simulink model "Integrated_Model"  (R2023b)
settings: Solver=ode23s  StartTime=0.0  StopTime=120  FixedStep=0.01  RelTol=1e-3
undefined symbols (not defined in the file): A_sm, A_stack, A_VGS_center, cmp, cp_coolant, ctrl, estNcr, eta_hex, eta_M, J_rotor, k_e_M, k_t_M, lambda, M_H2O, M_Nmix, M_O2, m_st_Nmix_init, m_st_O2_init, m_st_vp_init, p_amb, p_init, R_init, R_M, R_Nmix, R_O2, R_vp, RH_amb, T_amb, T_coolant, T_init, tbn, V_sm, V_stack, V_tbn_m, yO2_amb
libraries: slpidlib x5
(part 2 of 3)

== system Integrated_Model/SimpleFCstack/Calc_outlet_humidity ==
  note: ※凝縮が生じない場合の分圧比はモル分率に等しい
  RHin [-] : Inport
  Tin [K] : Inport  Port=2
  Tout [K] : Inport  Port=3
  pin [Pa] : Inport  Port=4
  pout [Pa] : Inport  Port=5
  Divide : Product  Inputs=*/
  Divide1 : Product  Inputs=*/
  MATLAB Function : MATLAB Function  TreatAsAtomicUnit=on
  MATLAB Function1 : MATLAB Function  TreatAsAtomicUnit=on
  Product : Product
  Product1 : Product
  Terminator : Terminator
  RHout [-] : Outport
  wires:
  MATLAB Function/1(psat) -> Product/2
  Tin [K]/1 -> MATLAB Function/1(Ts)
  Tout [K]/1 -> MATLAB Function1/1(Ts)
  RHin [-]/1 -> Product/1
  Product/1 -> Terminator/1, Divide/1  "pin,vp"
  pin [Pa]/1 -> Divide/2
  Divide/1 -> Product1/1  "pin,vp/pin"
  pout [Pa]/1 -> Product1/2
  Product1/1 -> Divide1/1  "pout,vp"
  MATLAB Function1/1(psat) -> Divide1/2
  Divide1/1 -> RHout [-]/1

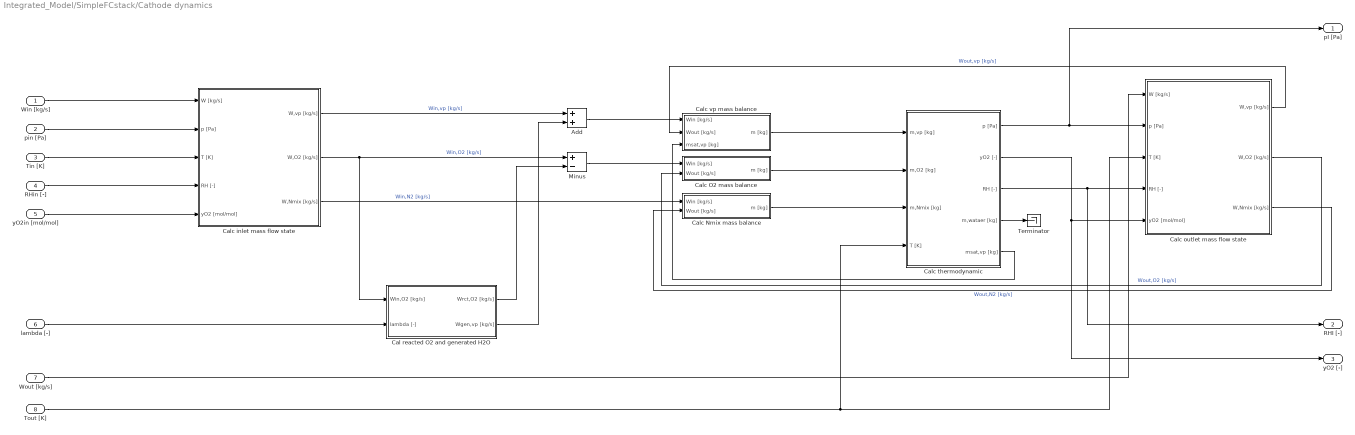
== system Integrated_Model/SimpleFCstack/Cathode dynamics ==
  Win [kg/s] : Inport
  pin [Pa] : Inport  Port=2
  Tin [K] : Inport  Port=3
  RHin [-] : Inport  Port=4
  yO2in [mol/mol] : Inport  Port=5
  lambda [-] : Inport  Port=6
  Wout [kg/s] : Inport  Port=7
  Tout [K] : Inport  Port=8
  Add : Sum
  Cal reacted O2 and generated H2O : Subsystem
  Calc Nmix mass balance : Subsystem
  Calc O2 mass balance : Subsystem
  Calc inlet mass flow state : Subsystem
  Calc outlet mass flow state : Subsystem
  Calc thermodynamic : Subsystem
  Calc vp mass balance : Subsystem
  Minus : Sum  Inputs=+-
  Terminator : Terminator
  pI [Pa] : Outport
  RHI [-] : Outport  Port=2
  yO2 [-] : Outport  Port=3
  wires:
  Calc outlet mass flow state/3(W,Nmix [kg/s]) -> Calc Nmix mass balance/2(Wout [kg/s])  "Wout,N2 [kg/s]"
  Calc vp mass balance/1(m [kg]) -> Calc thermodynamic/1(m,vp [kg])
  RHin [-]/1 -> Calc inlet mass flow state/4(RH [-])
  Calc outlet mass flow state/1(W,vp [kg/s]) -> Calc vp mass balance/2(Wout [kg/s])  "Wout,vp [kg/s]"
  Calc inlet mass flow state/2(W,O2 [kg/s]) -> Minus/1, Cal reacted O2 and generated H2O/1(Win,O2 [kg/s])  "Win,O2 [kg/s]"
  Win [kg/s]/1 -> Calc inlet mass flow state/1(W [kg/s])
  Calc O2 mass balance/1(m [kg]) -> Calc thermodynamic/2(m,O2 [kg])
  lambda [-]/1 -> Cal reacted O2 and generated H2O/2(lambda [-])
  Minus/1 -> Calc O2 mass balance/1(Win [kg/s])
  Calc thermodynamic/2(yO2 [-]) -> yO2 [-]/1, Calc outlet mass flow state/5(yO2 [mol/mol])
  Tout [K]/1 -> Calc outlet mass flow state/3(T [K]), Calc thermodynamic/4(T [K])
  Calc outlet mass flow state/2(W,O2 [kg/s]) -> Calc O2 mass balance/2(Wout [kg/s])  "Wout,O2 [kg/s]"
  Calc inlet mass flow state/3(W,Nmix [kg/s]) -> Calc Nmix mass balance/1(Win [kg/s])  "Win,N2 [kg/s]"
  Calc Nmix mass balance/1(m [kg]) -> Calc thermodynamic/3(m,Nmix [kg])
  Calc thermodynamic/3(RH [-]) -> RHI [-]/1, Calc outlet mass flow state/4(RH [-])
  Calc thermodynamic/1(p [Pa]) -> pI [Pa]/1, Calc outlet mass flow state/2(p [Pa])
  Calc thermodynamic/4(m,wataer [kg]) -> Terminator/1
  Cal reacted O2 and generated H2O/1(Wrct,O2 [kg/s]) -> Minus/2
  Calc thermodynamic/5(msat,vp [kg]) -> Calc vp mass balance/3(msat,vp [kg])
  Tin [K]/1 -> Calc inlet mass flow state/3(T [K])
  Calc inlet mass flow state/1(W,vp [kg/s]) -> Add/1  "Win,vp [kg/s]"
  Add/1 -> Calc vp mass balance/1(Win [kg/s])
  yO2in [mol/mol]/1 -> Calc inlet mass flow state/5(yO2 [mol/mol])
  Cal reacted O2 and generated H2O/2(Wgen,vp [kg/s]) -> Add/2
  pin [Pa]/1 -> Calc inlet mass flow state/2(p [Pa])
  Wout [kg/s]/1 -> Calc outlet mass flow state/1(W [kg/s])

== system Integrated_Model/SimpleFCstack/orifiece ==
  pin [Pa] : Inport
  pout [Pa] : Inport  Port=2
  Tin [K] : Inport  Port=3
  A_nzl [m^2] : Inport  Port=4
  R : Inport  Port=5
  kap : Inport  Port=6
  Constant2 : Constant  Value=Cd_nzl
  Divide1 : Product  Inputs=*/
  Product{,1..2,4} (4 alike) : Product
  Sqrt : Sqrt
  calc_phi : MATLAB Function  TreatAsAtomicUnit=on
  W [kg/s] : Outport
  wires:
  pout [Pa]/1 -> calc_phi/2(pout)
  pin [Pa]/1 -> calc_phi/1(pin), Divide1/1
  Tin [K]/1 -> Product/1
  A_nzl [m^2]/1 -> Product1/2
  R/1 -> Product/2
  Product/1 -> Sqrt/1
  Sqrt/1 -> Divide1/2
  Divide1/1 -> Product1/1
  kap/1 -> calc_phi/3(kap)
  calc_phi/1(phi) -> Product4/1
  Product1/1 -> Product4/2
  Product4/1 -> Product2/1
  Product2/1 -> W [kg/s]/1
  Constant2/1 -> Product2/2

== system Integrated_Model/SimpleTurbine/PowerCalculator ==
  Tin [K] : Inport
  Tout [K] : Inport  Port=2
  Win [kg/s] : Inport  Port=3
  cpin [J/kg*K] : Inport  Port=4
  eta_m [-] : Inport  Port=5
  omega [rad/s] : Inport  Port=6
  Divide3 : Product  Inputs=*/
  Minus : Sum  Inputs=+-
  Prevent division by zero : Subsystem
  Product1 : Product
  Product2 : Product
  Product6 : Product
  P_tbn [W] : Outport
  torque [Nm] : Outport  Port=2
  wires:
  Tout [K]/1 -> Minus/2
  Tin [K]/1 -> Minus/1
  Minus/1 -> Product2/1  "dT"
  Win [kg/s]/1 -> Product1/1
  cpin [J/kg*K]/1 -> Product1/2
  Product1/1 -> Product2/2  "W*cp"
  Product2/1 -> Product6/1
  eta_m [-]/1 -> Product6/2
  omega [rad/s]/1 -> Prevent division by zero/1(x)
  Divide3/1 -> torque [Nm]/1
  Product6/1 -> P_tbn [W]/1, Divide3/1  "P_tbn [W]"
  Prevent division by zero/1(x*) -> Divide3/2

== system Integrated_Model/SimpleTurbine/SimpleFlowCalculator(Orifice) ==
  pin [Pa] : Inport
  pout [Pa] : Inport  Port=2
  Tin [K] : Inport  Port=3
  A_VGS [m^2] : Inport  Port=4
  Rin : Inport  Port=5
  kapin : Inport  Port=6
  Divide1 : Product  Inputs=*/
  Product : Product
  Product1 : Product
  Product4 : Product
  Sqrt : Sqrt
  calc_phi : MATLAB Function  TreatAsAtomicUnit=on
  W [kg/s] : Outport
  wires:
  pin [Pa]/1 -> Divide1/1, calc_phi/1(pin)
  Divide1/1 -> Product1/1
  Product/1 -> Sqrt/1
  Product4/1 -> W [kg/s]/1
  calc_phi/1(phi) -> Product4/1
  A_VGS [m^2]/1 -> Product1/2
  Tin [K]/1 -> Product/1
  Sqrt/1 -> Divide1/2
  Rin/1 -> Product/2
  Product1/1 -> Product4/2
  pout [Pa]/1 -> calc_phi/2(pout)
  kapin/1 -> calc_phi/3(kap)

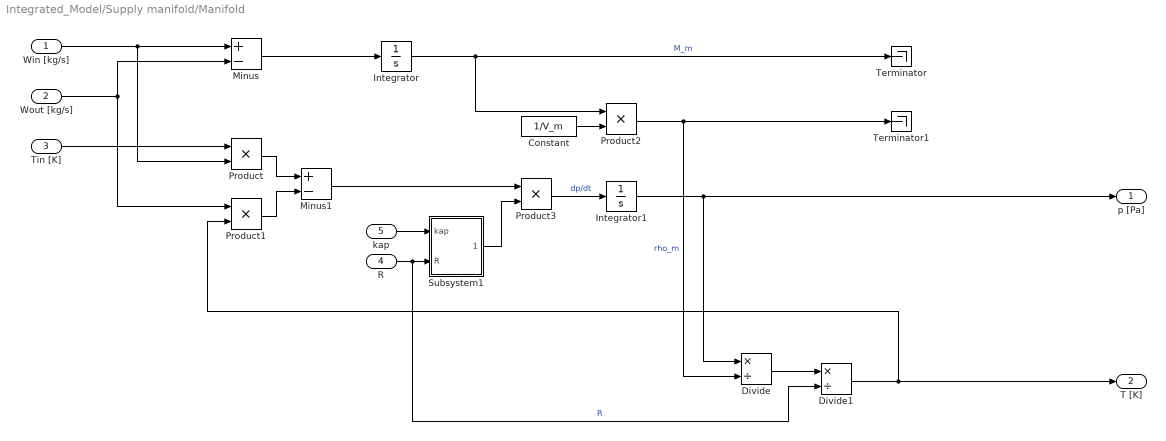
== system Integrated_Model/Supply manifold/Manifold ==
  Win [kg/s] : Inport
  Wout [kg/s] : Inport  Port=2
  Tin [K] : Inport  Port=3
  R : Inport  Port=4
  kap : Inport  Port=5
  Constant : Constant  Value=1/V_m
  Divide : Product  Inputs=*/
  Divide1 : Product  Inputs=*/
  Integrator : Integrator  InitialCondition=p_init*V_m/(R_init*T_init)
  Integrator1 : Integrator  InitialCondition=p_init
  Minus : Sum  Inputs=+-
  Minus1 : Sum  Inputs=+-
  Product{,1..3} (4 alike) : Product
  Subsystem1 : Subsystem
  Terminator : Terminator
  Terminator1 : Terminator
  p [Pa] : Outport
  T [K] : Outport  Port=2
  wires:
  Divide1/1 -> T [K]/1, Product1/2
  kap/1 -> Subsystem1/1(kap)
  Subsystem1/1(kap*R/V) -> Product3/2
  Constant/1 -> Product2/2
  Divide/1 -> Divide1/1
  Product/1 -> Minus1/1
  Minus/1 -> Integrator/1
  Integrator1/1 -> p [Pa]/1, Divide/1
  R/1 -> Divide1/2, Subsystem1/2(R)  "R"
  Product2/1 -> Terminator1/1, Divide/2  "rho_m"
  Wout [kg/s]/1 -> Product1/1, Minus/2
  Tin [K]/1 -> Product/1
  Product3/1 -> Integrator1/1  "dp/dt"
  Minus1/1 -> Product3/1
  Product1/1 -> Minus1/2
  Win [kg/s]/1 -> Minus/1, Product/2
  Integrator/1 -> Product2/1, Terminator/1  "M_m"

== system Integrated_Model/Supply manifold/Nozzle ==
  pin [Pa] : Inport
  pout [Pa] : Inport  Port=2
  Tin [K] : Inport  Port=3
  A_nzl [m^2] : Inport  Port=4
  R : Inport  Port=5
  kap : Inport  Port=6
  Constant2 : Constant  Value=Cd_nzl
  Divide1 : Product  Inputs=*/
  Product{,1..2,4} (4 alike) : Product
  Sqrt : Sqrt
  calc_phi : MATLAB Function  TreatAsAtomicUnit=on
  W [kg/s] : Outport
  wires:
  pout [Pa]/1 -> calc_phi/2(pout)
  pin [Pa]/1 -> calc_phi/1(pin), Divide1/1
  Tin [K]/1 -> Product/1
  A_nzl [m^2]/1 -> Product1/2
  R/1 -> Product/2
  Product/1 -> Sqrt/1
  Sqrt/1 -> Divide1/2
  Divide1/1 -> Product1/1
  kap/1 -> calc_phi/3(kap)
  calc_phi/1(phi) -> Product4/1
  Product1/1 -> Product4/2
  Product4/1 -> Product2/1
  Product2/1 -> W [kg/s]/1
  Constant2/1 -> Product2/2

== system Integrated_Model/Supply manifold/Subsystem ==
  note: ※凝縮が生じない場合の分圧比はモル分率に等しい
  RHin [-] : Inport
  Tin [K] : Inport  Port=2
  Tout [K] : Inport  Port=3
  pin [Pa] : Inport  Port=4
  pout [Pa] : Inport  Port=5
  Divide : Product  Inputs=*/
  Divide1 : Product  Inputs=*/
  MATLAB Function : MATLAB Function  TreatAsAtomicUnit=on
  MATLAB Function1 : MATLAB Function  TreatAsAtomicUnit=on
  Product : Product
  Product1 : Product
  Terminator : Terminator
  RHout [-] : Outport
  wires:
  MATLAB Function/1(psat) -> Product/2
  Tin [K]/1 -> MATLAB Function/1(Ts)
  Tout [K]/1 -> MATLAB Function1/1(Ts)
  RHin [-]/1 -> Product/1
  Product/1 -> Terminator/1, Divide/1  "pin,vp"
  pin [Pa]/1 -> Divide/2
  Divide/1 -> Product1/1  "pin,vp/pin"
  pout [Pa]/1 -> Product1/2
  Product1/1 -> Divide1/1  "pout,vp"
  MATLAB Function1/1(psat) -> Divide1/2
  Divide1/1 -> RHout [-]/1

== system Integrated_Model/Turbine Manifold/Subsystem1 ==
  In1 : Inport
  In2 : Inport  Port=2
  Constant : Constant  Value=1/V_m
  Product6 : Product  Inputs=3
  kap*R/V : Outport
  wires:
  In1/1 -> Product6/1
  Product6/1 -> kap*R/V/1
  In2/1 -> Product6/2
  Constant/1 -> Product6/3

== system Integrated_Model/Simple Compressor/cmpMAP/MUy ==
  pr_cmp : Inport
  Tin [K] : Inport  Port=2
  Uc [m/s] : Inport  Port=3
  Constant2 : Constant  Value=0.5
  Constant3 : Constant
  Divide : Product  Inputs=*/
  Minus : Sum  Inputs=+-
  Pow : Math  Operator=pow  RndMeth=Zero
  Prevent division by zero : Subsystem
  Product : Product
  Product1 : Product
  Product3 : Product
  Square : Math  Operator=square
  Subsystem1 : Subsystem
  MUy : Outport
  wires:
  Subsystem1/1((kap_cmp-1)/kap_cmp) -> Pow/2
  pr_cmp/1 -> Pow/1
  Tin [K]/1 -> Product/1
  [cp_cmp] -> Product/2
  Square/1 -> Product1/1
  Uc [m/s]/1 -> Square/1
  Constant2/1 -> Product1/2
  Constant3/1 -> Minus/2
  Pow/1 -> Minus/1
  Minus/1 -> Product3/1
  Product/1 -> Product3/2
  Product3/1 -> Divide/1
  Divide/1 -> MUy/1
  Product1/1 -> Prevent division by zero/1(x)
  Prevent division by zero/1(x*) -> Divide/2

== system Integrated_Model/Simple Compressor/cmpMAP/Subsystem ==
  MUy : Inport
  phi_max : Inport  Port=2
  beta : Inport  Port=3
  MUy_max : Inport  Port=4
  Constant : Constant
  Constant1 : Constant
  Divide : Product  Inputs=*/
  Exp : Math
  Minus : Sum  Inputs=+-
  Minus1 : Sum  Inputs=+-
  Product : Product
  Product1 : Product
  phi : Outport
  wires:
  MUy/1 -> Divide/1
  MUy_max/1 -> Divide/2
  Divide/1 -> Minus/1  "MUy/MUy_max"
  Constant/1 -> Minus/2
  Minus/1 -> Product/1
  Product/1 -> Exp/1
  beta/1 -> Product/2
  phi_max/1 -> Product1/2
  Product1/1 -> phi/1
  Exp/1 -> Minus1/2
  Constant1/1 -> Minus1/1
  Minus1/1 -> Product1/1

== system Integrated_Model/Simple Compressor/cmpMAP/Subsystem1 ==
  Product6 : Product
  kap*R : Outport
  wires:
  [kap_cmp] -> Product6/1
  Product6/1 -> kap*R/1
  [R_cmp] -> Product6/2

== system Integrated_Model/SimpleFCstack/Cathode dynamics/Cal reacted O2 and generated H2O ==
  Win,O2 [kg/s] : Inport
  lambda [-] : Inport  Port=2
  Constant1 : Constant  Value=M_O2
  Constant2 : Constant  Value=2
  Constant3 : Constant  Value=M_H2O
  Divide : Product  Inputs=*/
  Divide1 : Product  Inputs=*/  RndMeth=Zero  SaturateOnIntegerOverflow=on
  Product1 : Product
  Product2 : Product
  Wrct,O2 [kg/s] : Outport
  Wgen,vp [kg/s] : Outport  Port=2
  wires:
  Divide1/1 -> Wrct,O2 [kg/s]/1, Divide/1
  Win,O2 [kg/s]/1 -> Divide1/1
  Constant1/1 -> Divide/2
  Divide/1 -> Product1/1  "nrct,O2 [mol/s]"
  Constant2/1 -> Product1/2
  Product1/1 -> Product2/1  "ngen,vp [mol/s]"
  Constant3/1 -> Product2/2
  Product2/1 -> Wgen,vp [kg/s]/1
  lambda [-]/1 -> Divide1/2

== system Integrated_Model/SimpleFCstack/Cathode dynamics/Calc Nmix mass balance ==
  Win [kg/s] : Inport
  Wout [kg/s] : Inport  Port=2
  Integrator : Integrator  InitialCondition=m_st_Nmix_init
  Minus : Sum  Inputs=+-
  m [kg] : Outport
  wires:
  Win [kg/s]/1 -> Minus/1
  Wout [kg/s]/1 -> Minus/2
  Minus/1 -> Integrator/1
  Integrator/1 -> m [kg]/1

== system Integrated_Model/SimpleFCstack/Cathode dynamics/Calc O2 mass balance ==
  Win [kg/s] : Inport
  Wout [kg/s] : Inport  Port=2
  Integrator : Integrator  InitialCondition=m_st_O2_init
  Minus : Sum  Inputs=+-
  m [kg] : Outport
  wires:
  Integrator/1 -> m [kg]/1
  Minus/1 -> Integrator/1
  Wout [kg/s]/1 -> Minus/2
  Win [kg/s]/1 -> Minus/1

== system Integrated_Model/SimpleFCstack/Cathode dynamics/Calc inlet mass flow state ==
  W [kg/s] : Inport
  p [Pa] : Inport  Port=2
  T [K] : Inport  Port=3
  RH [-] : Inport  Port=4
  yO2 [mol/mol] : Inport  Port=5
  Add : Sum
  Calc absolute humidity ratio [kg/kgDA] : Subsystem
  Calc dry air (DA) properties : Subsystem
  Constant : Constant
  Constant1 : Constant
  Divide : Product  Inputs=*/
  Minus : Sum  Inputs=+-
  Minus1 : Sum  Inputs=+-
  Product : Product
  Product1 : Product
  W,vp [kg/s] : Outport
  W,O2 [kg/s] : Outport  Port=2
  W,Nmix [kg/s] : Outport  Port=3
  wires:
  p [Pa]/1 -> Calc absolute humidity ratio [kg/kgDA]/1(p [Pa])
  Calc dry air (DA) properties/2(xO2 [kg/kgDA]) -> Minus1/2, Product/2
  Calc absolute humidity ratio [kg/kgDA]/1(w [kg/kgDA]) -> Add/1  "win [kg/kgDA]"
  Calc dry air (DA) properties/1(M_DA [kg/mol]) -> Calc absolute humidity ratio [kg/kgDA]/4(M_DA [kg/mol])
  Product/1 -> W,O2 [kg/s]/1
  Divide/1 -> Minus/2, Product1/1, Product/1  "W,DA [kg/s]"
  Product1/1 -> W,Nmix [kg/s]/1
  Minus1/1 -> Product1/2
  Minus/1 -> W,vp [kg/s]/1
  yO2 [mol/mol]/1 -> Calc dry air (DA) properties/1(yO2)
  Constant1/1 -> Minus1/1
  RH [-]/1 -> Calc absolute humidity ratio [kg/kgDA]/3(RH [-])
  W [kg/s]/1 -> Minus/1, Divide/1
  Constant/1 -> Add/2
  Add/1 -> Divide/2  "1+w"
  T [K]/1 -> Calc absolute humidity ratio [kg/kgDA]/2(T [K])

== system Integrated_Model/SimpleFCstack/Cathode dynamics/Calc outlet mass flow state ==
  W [kg/s] : Inport
  p [Pa] : Inport  Port=2
  T [K] : Inport  Port=3
  RH [-] : Inport  Port=4
  yO2 [mol/mol] : Inport  Port=5
  Add : Sum
  Calc absolute humidity ratio [kg/kgDA] : Subsystem
  Calc dry air (DA) properties : Subsystem
  Constant : Constant
  Constant1 : Constant
  Divide : Product  Inputs=*/
  Minus : Sum  Inputs=+-
  Minus1 : Sum  Inputs=+-
  Product : Product
  Product1 : Product
  W,vp [kg/s] : Outport
  W,O2 [kg/s] : Outport  Port=2
  W,Nmix [kg/s] : Outport  Port=3
  wires:
  T [K]/1 -> Calc absolute humidity ratio [kg/kgDA]/2(T [K])
  Add/1 -> Divide/2  "1+w"
  Constant/1 -> Add/2
  W [kg/s]/1 -> Divide/1, Minus/1
  RH [-]/1 -> Calc absolute humidity ratio [kg/kgDA]/3(RH [-])
  Constant1/1 -> Minus1/1
  yO2 [mol/mol]/1 -> Calc dry air (DA) properties/1(yO2)
  Minus/1 -> W,vp [kg/s]/1
  Minus1/1 -> Product1/2
  Product1/1 -> W,Nmix [kg/s]/1
  Divide/1 -> Product/1, Product1/1, Minus/2  "W,DA [kg/s]"
  Product/1 -> W,O2 [kg/s]/1
  Calc dry air (DA) properties/1(M_DA [kg/mol]) -> Calc absolute humidity ratio [kg/kgDA]/4(M_DA [kg/mol])
  Calc absolute humidity ratio [kg/kgDA]/1(w [kg/kgDA]) -> Add/1  "win [kg/kgDA]"
  Calc dry air (DA) properties/2(xO2 [kg/kgDA]) -> Minus1/2, Product/2
  p [Pa]/1 -> Calc absolute humidity ratio [kg/kgDA]/1(p [Pa])

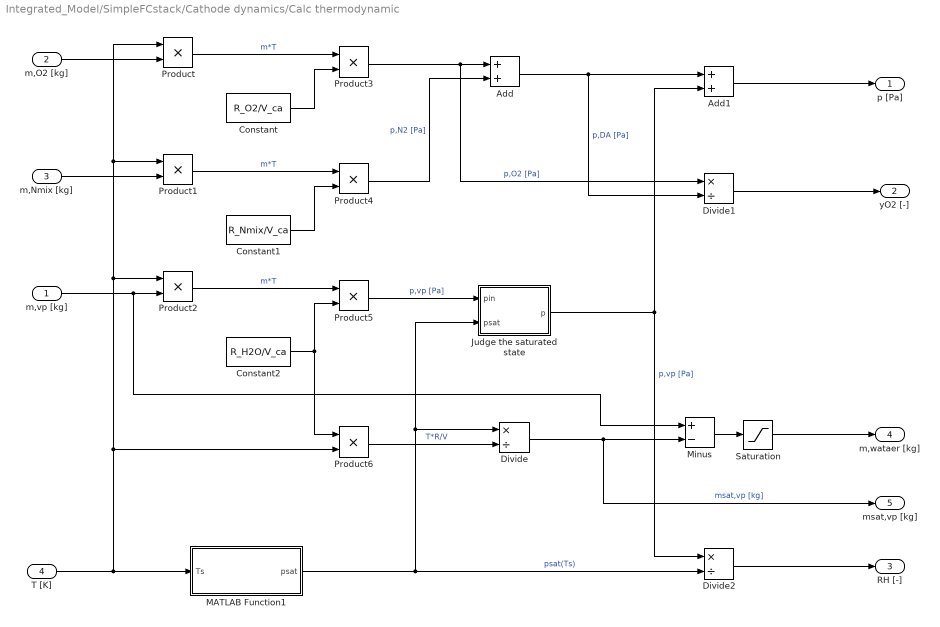
== system Integrated_Model/SimpleFCstack/Cathode dynamics/Calc thermodynamic ==
  m,vp [kg] : Inport
  m,O2 [kg] : Inport  Port=2
  m,Nmix [kg] : Inport  Port=3
  T [K] : Inport  Port=4
  Add : Sum
  Add1 : Sum
  Constant : Constant  Value=R_O2/V_ca
  Constant1 : Constant  Value=R_Nmix/V_ca
  Constant2 : Constant  Value=R_H2O/V_ca
  Divide : Product  Inputs=*/
  Divide1 : Product  Inputs=*/
  Divide2 : Product  Inputs=*/
  Judge the saturated state : MATLAB Function  TreatAsAtomicUnit=on
  MATLAB Function1 : MATLAB Function  TreatAsAtomicUnit=on
  Minus : Sum  Inputs=+-
  Product{,1..6} (7 alike) : Product
  Saturation : Saturate  UpperLimit=inf  LowerLimit=0
  p [Pa] : Outport
  yO2 [-] : Outport  Port=2
  RH [-] : Outport  Port=3
  m,wataer [kg] : Outport  Port=4
  msat,vp [kg] : Outport  Port=5
  wires:
  m,O2 [kg]/1 -> Product/2
  m,Nmix [kg]/1 -> Product1/2
  m,vp [kg]/1 -> Minus/1, Product2/2
  T [K]/1 -> MATLAB Function1/1(Ts), Product2/1, Product1/1, Product/1, Product6/2
  Product/1 -> Product3/1  "m*T"
  Product1/1 -> Product4/1  "m*T"
  Product2/1 -> Product5/1  "m*T"
  Constant/1 -> Product3/2
  Constant1/1 -> Product4/2
  Constant2/1 -> Product6/1, Product5/2
  Product5/1 -> Judge the saturated state/1(pin)  "p,vp [Pa]"
  MATLAB Function1/1(psat) -> Divide2/2, Divide/1, Judge the saturated state/2(psat)  "psat(Ts)"
  Product6/1 -> Divide/2  "T*R/V"
  Divide/1 -> msat,vp [kg]/1, Minus/2  "msat,vp [kg]"
  Product3/1 -> Divide1/1, Add/1  "p,O2 [Pa]"
  Product4/1 -> Add/2  "p,N2 [Pa]"
  Add/1 -> Add1/1, Divide1/2  "p,DA [Pa]"
  Divide1/1 -> yO2 [-]/1
  Add1/1 -> p [Pa]/1
  Judge the saturated state/1(p) -> Add1/2, Divide2/1  "p,vp [Pa]"
  Minus/1 -> Saturation/1
  Saturation/1 -> m,wataer [kg]/1
  Divide2/1 -> RH [-]/1

== system Integrated_Model/SimpleFCstack/Cathode dynamics/Calc vp mass balance ==
  note: 凝縮中は水蒸気量の質量は増えない
  note: 凝縮中に水蒸気量が減ると凝縮は起きなくなる
  Win [kg/s] : Inport
  Wout [kg/s] : Inport  Port=2
  msat,vp [kg] : Inport  Port=3
  Constant : Constant  Value=0
  Integrator : Integrator  InitialCondition=m_st_vp_init
  Judge the saturated state : MATLAB Function  TreatAsAtomicUnit=on
  Minus : Sum  Inputs=+-
  Scope{,1..3} (4 alike) : Scope
  Switch : Switch  Criteria=u2 > Threshold  SaturateOnIntegerOverflow=off  InputSameDT=off
  Switch1 : Switch  Criteria=u2 > Threshold  SaturateOnIntegerOverflow=off  InputSameDT=off
  m [kg] : Outport
  wires:
  Win [kg/s]/1 -> Minus/1
  Wout [kg/s]/1 -> Minus/2
  [cnd_flag] -> Switch/2
  Minus/1 -> Scope1/1, Switch1/2, Switch1/3, Switch/3
  Switch/1 -> Integrator/1
  Integrator/1 -> Judge the saturated state/1(m), Scope/1, m [kg]/1
  msat,vp [kg]/1 -> Judge the saturated state/2(msat)
  Constant/1 -> Switch1/1
  Judge the saturated state/1(flg) -> Scope3/1, [cnd_flag]
  Switch1/1 -> Switch/1, Scope2/1

== system Integrated_Model/SimpleTurbine/PowerCalculator/Prevent division by zero ==
  note: ※ゼロ除算防止 : x* = sqrt(x^2 + xth^2)
  x : Inport
  Add : Sum
  Constant4 : Constant  Value=0.01^2
  Sqrt : Sqrt
  Square1 : Math  Operator=square
  x* : Outport
  wires:
  Constant4/1 -> Add/2
  Square1/1 -> Add/1
  x/1 -> Square1/1
  Add/1 -> Sqrt/1
  Sqrt/1 -> x*/1

== system Integrated_Model/Supply manifold/Manifold/Subsystem1 ==
  kap : Inport
  R : Inport  Port=2
  Constant : Constant  Value=1/V_m
  Product6 : Product  Inputs=3
  kap*R/V : Outport
  wires:
  kap/1 -> Product6/1
  Product6/1 -> kap*R/V/1
  R/1 -> Product6/2
  Constant/1 -> Product6/3

== system Integrated_Model/Simple Compressor/cmpMAP/MUy/Prevent division by zero ==
  note: ※ゼロ除算防止 : x* = sqrt(x^2 + xth^2)
  x : Inport
  Add : Sum
  Constant4 : Constant  Value=0.01^2
  Sqrt : Sqrt
  Square1 : Math  Operator=square
  x* : Outport
  wires:
  Constant4/1 -> Add/2
  Square1/1 -> Add/1
  x/1 -> Square1/1
  Add/1 -> Sqrt/1
  Sqrt/1 -> x*/1

== system Integrated_Model/Simple Compressor/cmpMAP/MUy/Subsystem1 ==
  Constant5 : Constant
  Divide4 : Product  Inputs=*/
  Minus1 : Sum  Inputs=+-
  (kap_cmp-1)/kap_cmp : Outport
  wires:
  [kap_cmp] -> Divide4/2, Minus1/1
  Divide4/1 -> (kap_cmp-1)/kap_cmp/1
  Constant5/1 -> Minus1/2
  Minus1/1 -> Divide4/1

== system Integrated_Model/SimpleFCstack/Cathode dynamics/Calc inlet mass flow state/Calc absolute humidity ratio [kg//kgDA] ==
  p [Pa] : Inport
  T [K] : Inport  Port=2
  RH [-] : Inport  Port=3
  M_DA [kg/mol] : Inport  Port=4
  Constant : Constant  Value=M_H2O
  Divide : Product  Inputs=*/
  Divide1 : Product  Inputs=*/
  MATLAB Function1 : MATLAB Function  TreatAsAtomicUnit=on
  Minus : Sum  Inputs=+-
  Product : Product
  Product1 : Product
  w [kg/kgDA] : Outport
  wires:
  T [K]/1 -> MATLAB Function1/1(Ts)
  Minus/1 -> Divide/2  "p,DA"
  Product/1 -> Divide/1, Minus/2  "p,vp"
  Divide1/1 -> Product1/2
  RH [-]/1 -> Product/2
  M_DA [kg/mol]/1 -> Divide1/2
  Constant/1 -> Divide1/1
  Product1/1 -> w [kg/kgDA]/1
  MATLAB Function1/1(psat) -> Product/1  "psat(Ts)"
  Divide/1 -> Product1/1
  p [Pa]/1 -> Minus/1

== system Integrated_Model/SimpleFCstack/Cathode dynamics/Calc inlet mass flow state/Calc dry air (DA) properties ==
  yO2 : Inport
  Add1 : Sum
  Constant1 : Constant  Value=M_O2
  Constant2 : Constant
  Constant3 : Constant  Value=M_Nmix
  Divide : Product  Inputs=*/
  Minus : Sum  Inputs=+-
  Product : Product
  Product1 : Product
  M_DA [kg/mol] : Outport
  xO2 [kg/kgDA] : Outport  Port=2
  wires:
  Product/1 -> Divide/1, Add1/1  "m_O2 [kg/molDA]"
  Constant2/1 -> Minus/1
  Constant3/1 -> Product1/1
  Minus/1 -> Product1/2  "1-yO2"
  yO2/1 -> Minus/2, Product/2
  Add1/1 -> M_DA [kg/mol]/1, Divide/2  "M_DA [kg/mol]"
  Constant1/1 -> Product/1
  Product1/1 -> Add1/2
  Divide/1 -> xO2 [kg/kgDA]/1

== system Integrated_Model/SimpleFCstack/Cathode dynamics/Calc outlet mass flow state/Calc absolute humidity ratio [kg//kgDA] ==
  p [Pa] : Inport
  T [K] : Inport  Port=2
  RH [-] : Inport  Port=3
  M_DA [kg/mol] : Inport  Port=4
  Constant : Constant  Value=M_H2O
  Divide : Product  Inputs=*/
  Divide1 : Product  Inputs=*/
  MATLAB Function1 : MATLAB Function  TreatAsAtomicUnit=on
  Minus : Sum  Inputs=+-
  Product : Product
  Product1 : Product
  w [kg/kgDA] : Outport
  wires:
  p [Pa]/1 -> Minus/1
  Divide/1 -> Product1/1
  MATLAB Function1/1(psat) -> Product/1  "psat(Ts)"
  Product1/1 -> w [kg/kgDA]/1
  Constant/1 -> Divide1/1
  M_DA [kg/mol]/1 -> Divide1/2
  RH [-]/1 -> Product/2
  Divide1/1 -> Product1/2
  Product/1 -> Minus/2, Divide/1  "p,vp"
  Minus/1 -> Divide/2  "p,DA"
  T [K]/1 -> MATLAB Function1/1(Ts)

== system Integrated_Model/SimpleFCstack/Cathode dynamics/Calc outlet mass flow state/Calc dry air (DA) properties ==
  yO2 : Inport
  Add1 : Sum
  Constant1 : Constant  Value=M_O2
  Constant2 : Constant
  Constant3 : Constant  Value=M_Nmix
  Divide : Product  Inputs=*/
  Minus : Sum  Inputs=+-
  Product : Product
  Product1 : Product
  M_DA [kg/mol] : Outport
  xO2 [kg/kgDA] : Outport  Port=2
  wires:
  Divide/1 -> xO2 [kg/kgDA]/1
  Product1/1 -> Add1/2
  Constant1/1 -> Product/1
  Add1/1 -> Divide/2, M_DA [kg/mol]/1  "M_DA [kg/mol]"
  yO2/1 -> Product/2, Minus/2
  Minus/1 -> Product1/2  "1-yO2"
  Constant3/1 -> Product1/1
  Constant2/1 -> Minus/1
  Product/1 -> Add1/1, Divide/1  "m_O2 [kg/molDA]"

== matlab function Integrated_Model/SimpleFCstack/Cathode dynamics/Calc thermodynamic/Judge the saturated state ==
  data: pin input; p output; psat input
function p = fcn(pin,psat)
    if pin < psat
        p = pin;
    else
        p = psat;  
    end
end

== matlab function Integrated_Model/SimpleFCstack/Cathode dynamics/Calc thermodynamic/MATLAB Function1 ==
  data: Ts input; psat output
function psat = sat_vp_pressure(Ts)
    P_CONVERT = 0.001;
    C1 = -5.6745359e3;
    C2 = 6.3925247;
    C3 = -9.6778430e-3;
    C4 = 6.2215701e-7;
    C5 = 2.0747825e-9;
    C6 = -9.4840240e-13;
    C7 = 4.1635019;
    N1 = 0.11670521452767e4;
    N2 = -0.72421316703206e6;
    N3 = -0.17073846940092e2;
    N4 = 0.12020824702470e5;
    N5 = -0.32325550322333e7;
    N6 = 0.14915108613530e2;
    N7 = -0.4823265731591e4;
    N8 = 0.40511340542057e6;
    N9 = -0.23855557567849e0;
    N10 = 0.65017534844798e3;
    
    if Ts < 273.15+0.01
        % -100~0.01C//三重点を計算以下は wexler-hyland のシミュレーションプログラム式
        psat = exp(C1 / Ts + C2 + C3 * Ts + C4 * Ts^2 + C5 * Ts^3 + C6 * Ts^4 + C7 * log(Ts)) * P_CONVERT;
    else
        %　~647.096K//臨界温度まで一定とするは IAPWS-IF97 実用国際状態式
        alpha = Ts + N9 / (Ts - N10);
        a2 = alpha * alpha;
        A = a2 + N1 * alpha + N2;
        B = N3 * a2 + N4 * alpha + N5;
        C = N6 * a2 + N7 * alpha + N8;
        psat = (2 * C / (-B + (B * B - 4 * A * C)^0.5))^4 / P_CONVERT;
    end 
    psat = psat*1000; %kPa to Pa
end

== matlab function Integrated_Model/SimpleFCstack/Cathode dynamics/Calc vp mass balance/Judge the saturated state ==
  data: m input; flg output; msat input
function flg = fcn(m,msat)
    if m < msat
        flg = 0;
    else
        flg = 1;  
    end
end

== matlab function Integrated_Model/SimpleFCstack/MATLAB Function ==
  data: p input; T input; RH input; yO2 input; M output; R output; cp output; kap output; M_Nmix parameter; M_H2O parameter; M_O2 parameter
%% 湿り空気の状態量計算
function [M, R, cp, kap] = calc_MA_property(p, T, RH, yO2, M_Nmix, M_H2O, M_O2)
    % 湿り空気の物性値計算
    gsprop = GasProperties;
    [M,R,cp,kap] = gsprop.getMAprop(p, T, RH, yO2);
end

%% Calculate saturated vapor pressure [Pa]
function psat = sat_vp_pressure(Ts)
    P_CONVERT = 0.001;
    C1 = -5.6745359e3;
    C2 = 6.3925247;
    C3 = -9.6778430e-3;
    C4 = 6.2215701e-7;
    C5 = 2.0747825e-9;
    C6 = -9.4840240e-13;
    C7 = 4.1635019;
    N1 = 0.11670521452767e4;
    N2 = -0.72421316703206e6;
    N3 = -0.17073846940092e2;
    N4 = 0.12020824702470e5;
    N5 = -0.32325550322333e7;
    N6 = 0.14915108613530e2;
    N7 = -0.4823265731591e4;
    N8 = 0.40511340542057e6;
    N9 = -0.23855557567849e0;
    N10 = 0.65017534844798e3;
    
    if Ts < 273.15+0.01
        % -100~0.01C//三重点を計算以下は wexler-hyland のシミュレーションプログラム式
        psat = exp(C1 / Ts + C2 + C3 * Ts + C4 * Ts^2 + C5 * Ts^3 + C6 * Ts^4 + C7 * log(Ts)) * P_CONVERT;
    else
        %　~647.096K//臨界温度まで一定とするは IAPWS-IF97 実用国際状態式
        alpha = Ts + N9 / (Ts - N10);
        a2 = alpha * alpha;
        A = a2 + N1 * alpha + N2;
        B = N3 * a2 + N4 * alpha + N5;
        C = N6 * a2 + N7 * alpha + N8;
        psat = (2 * C / (-B + (B * B - 4 * A * C)^0.5))^4 / P_CONVERT;
    end 
    psat = psat*1000; %kPa to Pa
end

== matlab function Integrated_Model/SimpleHumidifire_std/calc_hm_dry ==
  data: W_in input; W_out output; p_in input; T_in input; RH_in input; yO2_in input; W_vp_inj input; p_out output; T_out output; RH_out output; yO2_out output; M_O2 parameter; M_Nmix parameter; M_H2O parameter
%% 加湿／除湿計算
function [W_out, p_out, T_out, RH_out, yO2_out] = HM_std(W_in, p_in, T_in, RH_in, yO2_in, W_vp_inj, M_O2, M_Nmix, M_H2O)
    % 湿り空気の状態計算
    [W_O2_in, W_N2_in, W_vp_in, p_O2_in, p_N2_in, p_vp_in, M_in, R_in, cp_in, kap_in] = calc_MA_property(W_in, p_in, T_in, RH_in, yO2_in, M_O2, M_Nmix, M_H2O);

    % 水蒸気の注入
    W_vp_out = W_vp_in + W_vp_inj;  % [kg/s]

    % 出口流量計算
    W_O2_out = W_O2_in; % [kg/s]
    W_N2_out = W_N2_in; % [kg/s]
    W_out = W_O2_out + W_N2_out + W_vp_out; % [kg/s]

    % 出口圧計算

    % 出口全圧は一定とする
    p_out = p_in;
    ndot_O2_out = W_O2_out/M_O2;
    ndot_N2_out = W_N2_out/M_Nmix;
    ndot_vp_out = W_vp_out/M_H2O;
    
    if W_vp_out <= 0
        p_vp_out = 0;
    else
        p_vp_out = ndot_vp_out/(ndot_O2_out+ndot_N2_out+ndot_vp_out)*p_out;  % [Pa]
    end

    % 温度は一定とする
    T_out = T_in;       % [K]

    % 相対湿度計算
    RH_out = p_vp_out/sat_vp_pressure(T_out);

    % 空気組成は一定とする
    yO2_out = yO2_in;   % [-]
end

%% 湿り空気の状態量計算
function [W_O2, W_N2, W_vp, p_O2, p_N2, p_vp, M, R, cp, kap] = calc_MA_property(W, p, T, RH, yO2, M_O2, M_Nmix, M_vp)
    % 湿り空気の物性値計算
    gsprop = GasProperties;
    [M,R,cp,kap] = gsprop.getMAprop(p, T, RH, yO2);

    % 分圧計算
    p_vp_sat = sat_vp_pressure(T);
    p_vp = RH * p_vp_sat;
    p_DA = p - p_vp;
    p_O2 = yO2 * p_DA;
    p_N2 = p_DA - p_O2;
    
    % 湿り空気のモル分率計算
    x_O2 = p_O2/p;
    x_N2 = p_N2/p;
    x_vp = p_vp/p;

    % 質量分率計算
    w_O2 = x_O2*M_O2 / M;
    w_N2 = x_N2*M_Nmix / M;
    w_vp = x_vp*M_vp / M;

    % 各分子の質量流量
    W_O2 = W * w_O2;    % [kg/s]
    W_N2 = W * w_N2;    % [kg/s]
    W_vp = W * w_vp;    % [kg/s]

end

%% Calculate saturated vapor pressure [Pa]
function psat = sat_vp_pressure(Ts)
    P_CONVERT = 0.001;
    C1 = -5.6745359e3;
    C2 = 6.3925247;
    C3 = -9.6778430e-3;
    C4 = 6.2215701e-7;
    C5 = 2.0747825e-9;
    C6 = -9.4840240e-13;
    C7 = 4.1635019;
    N1 = 0.11670521452767e4;
    N2 = -0.72421316703206e6;
    N3 = -0.17073846940092e2;
    N4 = 0.12020824702470e5;
    N5 = -0.32325550322333e7;
    N6 = 0.14915108613530e2;
    N7 = -0.4823265731591e4;
    N8 = 0.40511340542057e6;
    N9 = -0.23855557567849e0;
    N10 = 0.65017534844798e3;
    
    if Ts < 273.15+0.01
        % -100~0.01C//三重点を計算以下は wexler-hyland のシミュレーションプログラム式
        psat = exp(C1 / Ts + C2 + C3 * Ts + C4 * Ts^2 + C5 * Ts^3 + C6 * Ts^4 + C7 * log(Ts)) * P_CONVERT;
    else
        %　~647.096K//臨界温度まで一定とするは IAPWS-IF97 実用国際状態式
        alpha = Ts + N9 / (Ts - N10);
        a2 = alpha * alpha;
        A = a2 + N1 * alpha + N2;
        B = N3 * a2 + N4 * alpha + N5;
        C = N6 * a2 + N7 * alpha + N8;
        psat = (2 * C / (-B + (B * B - 4 * A * C)^0.5))^4 / P_CONVERT;
    end 
    psat = psat*1000; %kPa to Pa
end

== matlab function Integrated_Model/SimpleHumidifire_std/calc_hm_W_vp_inj ==
  data: W_in_dry input; W_vp_inj_ctrl output; p_in_dry input; T_in_dry input; RH_in_dry input; yO2_in_dry input; W_in_wet input; p_in_wet input; T_in_wet input; RH_in_wet input; yO2_in_wet input; RH_out_dry_tar input; M_O2 parameter; M_Nmix parameter; M_H2O parameter
%% 水交換制御量の計算
function W_vp_inj_ctrl = calc_W_vp_inj_ctrl(W_in_dry, p_in_dry, T_in_dry, RH_in_dry, yO2_in_dry,W_in_wet, p_in_wet, T_in_wet, RH_in_wet, yO2_in_wet,RH_out_dry_tar, M_O2, M_Nmix, M_H2O)
    % 物理定数の定義

    % 湿り空気の分圧計算
    % DRY側
    [W_O2_in_dry, W_N2_in_dry, W_vp_in_dry, p_O2_in_dry, p_N2_in_dry, p_vp_in_dry, M_in_dry, R_in_dry, cp_in_dry, kap_in_dry] = calc_MA_property(W_in_dry, p_in_dry, T_in_dry, RH_in_dry, yO2_in_dry, M_O2, M_Nmix, M_H2O);
    % WET側
    [W_O2_in_wet, W_N2_in_wet, W_vp_in_wet, p_O2_in_wet, p_N2_in_wet, p_vp_in_wet, M_in_wet, R_in_wet, cp_in_wet, kap_in_wet] = calc_MA_property(W_in_wet, p_in_wet, T_in_wet, RH_in_wet, yO2_in_wet, M_O2, M_Nmix, M_H2O);

    % DRY側の出口空気湿度をRH_out_dry_tarにする水蒸気注入量を計算
    % 入口モル流量の計算
    ndot_O2_in_dry = W_O2_in_dry/M_O2;
    ndot_N2_in_dry = W_N2_in_dry/M_Nmix;
    % 目標湿度における水蒸気分圧 (温度一定と仮定する)
    p_vp_out_dry_tar = RH_out_dry_tar * sat_vp_pressure(T_in_dry);
    % 水蒸気注入量を計算 (圧力一定と仮定する)
    W_vp_inj_ctrl_dry =  M_H2O * (ndot_O2_in_dry + ndot_N2_in_dry) * p_vp_out_dry_tar /(p_in_dry - p_vp_out_dry_tar) - W_vp_in_dry;

    % WET側と交換可能な水蒸気量の上限値を計算
    W_vp_inj_lim_wet =  W_vp_in_wet - 0;

    % 小さいほうが交換可能な水蒸気量となる
    W_vp_inj_ctrl = min(W_vp_inj_ctrl_dry, W_vp_inj_lim_wet);
end

%% 湿り空気の状態量計算
function [W_O2, W_N2, W_vp, p_O2, p_N2, p_vp, M, R, cp, kap] = calc_MA_property(W, p, T, RH, yO2, M_O2, M_Nmix, M_vp)
    % 湿り空気の物性値計算
    gsprop = GasProperties;
    [M,R,cp,kap] = gsprop.getMAprop(p, T, RH, yO2);

    % 分圧計算
    p_vp_sat = sat_vp_pressure(T);
    p_vp = RH * p_vp_sat;
    p_DA = p - p_vp;
    p_O2 = yO2 * p_DA;
    p_N2 = p_DA - p_O2;
    
    % 湿り空気のモル分率計算
    x_O2 = p_O2/p;
    x_Nmix = p_N2/p;
    x_vp = p_vp/p;

    % 質量分率計算
    w_O2 = x_O2*M_O2 / M;
    w_N2 = x_Nmix*M_Nmix / M;
    w_vp = x_vp*M_vp / M;

    % 各分子の質量流量
    W_O2 = W * w_O2;    % [kg/s]
    W_N2 = W * w_N2;    % [kg/s]
    W_vp = W * w_vp;    % [kg/s]
end

%% Calculate saturated vapor pressure [Pa]
function psat = sat_vp_pressure(Ts)
    P_CONVERT = 0.001;
    C1 = -5.6745359e3;
    C2 = 6.3925247;
    C3 = -9.6778430e-3;
    C4 = 6.2215701e-7;
    C5 = 2.0747825e-9;
    C6 = -9.4840240e-13;
    C7 = 4.1635019;
    N1 = 0.11670521452767e4;
    N2 = -0.72421316703206e6;
    N3 = -0.17073846940092e2;
    N4 = 0.12020824702470e5;
    N5 = -0.32325550322333e7;
    N6 = 0.14915108613530e2;
    N7 = -0.4823265731591e4;
    N8 = 0.40511340542057e6;
    N9 = -0.23855557567849e0;
    N10 = 0.65017534844798e3;
    
    if Ts < 273.15+0.01
        % -100~0.01C//三重点を計算以下は wexler-hyland のシミュレーションプログラム式
        psat = exp(C1 / Ts + C2 + C3 * Ts + C4 * Ts^2 + C5 * Ts^3 + C6 * Ts^4 + C7 * log(Ts)) * P_CONVERT;
    else
        %　~647.096K//臨界温度まで一定とするは IAPWS-IF97 実用国際状態式
        alpha = Ts + N9 / (Ts - N10);
        a2 = alpha * alpha;
        A = a2 + N1 * alpha + N2;
        B = N3 * a2 + N4 * alpha + N5;
        C = N6 * a2 + N7 * alpha + N8;
        psat = (2 * C / (-B + (B * B - 4 * A * C)^0.5))^4 / P_CONVERT;
    end 
    psat = psat*1000; %kPa to Pa
end

== matlab function Integrated_Model/SimpleHumidifire_std/calc_hm_wet ==
  data: W_in input; W_out output; p_in input; T_in input; RH_in input; yO2_in input; W_vp_inj input; p_out output; T_out output; RH_out output; yO2_out output; M_O2 parameter; M_Nmix parameter; M_H2O parameter
%% 加湿／除湿計算
function [W_out, p_out, T_out, RH_out, yO2_out] = HM_std(W_in, p_in, T_in, RH_in, yO2_in, W_vp_inj, M_O2, M_Nmix, M_H2O)
    % 湿り空気の状態計算
    [W_O2_in, W_N2_in, W_vp_in, p_O2_in, p_N2_in, p_vp_in, M_in, R_in, cp_in, kap_in] = calc_MA_property(W_in, p_in, T_in, RH_in, yO2_in, M_O2, M_Nmix, M_H2O);

    % 水蒸気の注入
    W_vp_out = W_vp_in + W_vp_inj;  % [kg/s]

    % 出口流量計算
    W_O2_out = W_O2_in; % [kg/s]
    W_N2_out = W_N2_in; % [kg/s]
    W_out = W_O2_out + W_N2_out + W_vp_out; % [kg/s]

    % 出口圧計算

    % 出口全圧は一定とする
    p_out = p_in;
    ndot_O2_out = W_O2_out/M_O2;
    ndot_N2_out = W_N2_out/M_Nmix;
    ndot_vp_out = W_vp_out/M_H2O;
    
    if W_vp_out <= 0
        p_vp_out = 0;
    else
        p_vp_out = ndot_vp_out/(ndot_O2_out+ndot_N2_out+ndot_vp_out)*p_out;  % [Pa]
    end

    % 温度は一定とする
    T_out = T_in;       % [K]

    % 相対湿度計算
    RH_out = p_vp_out/sat_vp_pressure(T_out);

    % 空気組成は一定とする
    yO2_out = yO2_in;   % [-]
end

%% 湿り空気の状態量計算
function [W_O2, W_N2, W_vp, p_O2, p_N2, p_vp, M, R, cp, kap] = calc_MA_property(W, p, T, RH, yO2, M_O2, M_Nmix, M_vp)
    % 湿り空気の物性値計算
    gsprop = GasProperties;
    [M,R,cp,kap] = gsprop.getMAprop(p, T, RH, yO2);

    % 分圧計算
    p_vp_sat = sat_vp_pressure(T);
    p_vp = RH * p_vp_sat;
    p_DA = p - p_vp;
    p_O2 = yO2 * p_DA;
    p_N2 = p_DA - p_O2;
    
    % 湿り空気のモル分率計算
    x_O2 = p_O2/p;
    x_N2 = p_N2/p;
    x_vp = p_vp/p;

    % 質量分率計算
    w_O2 = x_O2*M_O2 / M;
    w_N2 = x_N2*M_Nmix / M;
    w_vp = x_vp*M_vp / M;

    % 各分子の質量流量
    W_O2 = W * w_O2;    % [kg/s]
    W_N2 = W * w_N2;    % [kg/s]
    W_vp = W * w_vp;    % [kg/s]

end

%% Calculate saturated vapor pressure [Pa]
function psat = sat_vp_pressure(Ts)
    P_CONVERT = 0.001;
    C1 = -5.6745359e3;
    C2 = 6.3925247;
    C3 = -9.6778430e-3;
    C4 = 6.2215701e-7;
    C5 = 2.0747825e-9;
    C6 = -9.4840240e-13;
    C7 = 4.1635019;
    N1 = 0.11670521452767e4;
    N2 = -0.72421316703206e6;
    N3 = -0.17073846940092e2;
    N4 = 0.12020824702470e5;
    N5 = -0.32325550322333e7;
    N6 = 0.14915108613530e2;
    N7 = -0.4823265731591e4;
    N8 = 0.40511340542057e6;
    N9 = -0.23855557567849e0;
    N10 = 0.65017534844798e3;
    
    if Ts < 273.15+0.01
        % -100~0.01C//三重点を計算以下は wexler-hyland のシミュレーションプログラム式
        psat = exp(C1 / Ts + C2 + C3 * Ts + C4 * Ts^2 + C5 * Ts^3 + C6 * Ts^4 + C7 * log(Ts)) * P_CONVERT;
    else
        %　~647.096K//臨界温度まで一定とするは IAPWS-IF97 実用国際状態式
        alpha = Ts + N9 / (Ts - N10);
        a2 = alpha * alpha;
        A = a2 + N1 * alpha + N2;
        B = N3 * a2 + N4 * alpha + N5;
        C = N6 * a2 + N7 * alpha + N8;
        psat = (2 * C / (-B + (B * B - 4 * A * C)^0.5))^4 / P_CONVERT;
    end 
    psat = psat*1000; %kPa to Pa
end

== matlab function Integrated_Model/SimpleHEX_std/MATLAB Function ==
  data: W_in input; W_out output; p_in input; T_in input; RH_in input; yO2_in input; W_cool input; p_out output; T_out output; RH_out output; yO2_out output; T_cool input; cp_cool input; eta_hex input; M_O2 parameter; M_Nmix parameter; M_H2O parameter
%% 伝熱計算
function [W_out, p_out, T_out, RH_out, yO2_out] = HEX_std(W_in, p_in, T_in, RH_in, yO2_in, W_cool, T_cool, cp_cool, eta_hex, M_O2, M_Nmix, M_H2O)
    % 湿り空気の状態計算
    [W_O2_in, W_N2_in, W_vp_in, p_O2_in, p_N2_in, p_vp_in, M_in, R_in, cp_in, kap_in] = calc_MA_property(W_in, p_in, T_in, RH_in, yO2_in, M_O2, M_Nmix, M_H2O);

    % 熱容量の計算
    C_hot  = cp_in * W_in;
    C_cold = cp_cool * W_cool;
    C_min = min(C_hot,C_cold);
    % 熱交換量計算
    Q_hex = eta_hex * C_min*(T_in - T_cool);

    % 出口温度の計算
    if W_in <= 0
        T_out = T_in;
    else
        T_out = T_in - Q_hex/(cp_in*W_in);
    end

    % 相対湿度計算
    RH_out = p_vp_in/sat_vp_pressure(T_out);
    if RH_out < 1
        % 流量は一定とする
        W_out = W_in;       % [kg/s]
        % 圧力は一定とする
        p_out = p_in;       % [Pa]
    else
        RH_out = 1;
        % 凝縮した分の減圧量を加味
        p_vp_out = sat_vp_pressure(T_out);
        p_out = p_O2_in + p_N2_in + p_vp_out;
        % 凝縮した分の流量減少を加味
        p_vp_out = sat_vp_pressure(T_out);
        if p_vp_in <= 0
            W_vp_out = 0;
        else
            W_vp_out = p_vp_out/p_vp_in * W_vp_in;
        end
        W_out = W_O2_in + W_N2_in + W_vp_out;

    end

    % 空気組成は一定とする
    yO2_out = yO2_in;   % [-]
end


%% 湿り空気の状態量計算
function [W_O2, W_N2, W_vp, p_O2, p_N2, p_vp, M, R, cp, kap] = calc_MA_property(W, p, T, RH, yO2, M_O2, M_Nmix, M_vp)
    % 湿り空気の物性値計算
    gsprop = GasProperties;
    [M,R,cp,kap] = gsprop.getMAprop(p, T, RH, yO2);

    % 分圧計算
    p_vp_sat = sat_vp_pressure(T);
    p_vp = RH * p_vp_sat;
    p_DA = p - p_vp;
    p_O2 = yO2 * p_DA;
    p_N2 = p_DA - p_O2;
    
    % 湿り空気のモル分率計算
    x_O2 = p_O2/p;
    x_Nmix = p_N2/p;
    x_vp = p_vp/p;

    % 質量分率計算
    w_O2 = x_O2*M_O2 / M;
    w_N2 = x_Nmix*M_Nmix / M;
    w_vp = x_vp*M_vp / M;

    % 各分子の質量流量
    W_O2 = W * w_O2;    % [kg/s]
    W_N2 = W * w_N2;    % [kg/s]
    W_vp = W * w_vp;    % [kg/s]
end

%% Calculate saturated vapor pressure [Pa]
function psat = sat_vp_pressure(Ts)
    P_CONVERT = 0.001;
    C1 = -5.6745359e3;
    C2 = 6.3925247;
    C3 = -9.6778430e-3;
    C4 = 6.2215701e-7;
    C5 = 2.0747825e-9;
    C6 = -9.4840240e-13;
    C7 = 4.1635019;
    N1 = 0.11670521452767e4;
    N2 = -0.72421316703206e6;
    N3 = -0.17073846940092e2;
    N4 = 0.12020824702470e5;
    N5 = -0.32325550322333e7;
    N6 = 0.14915108613530e2;
    N7 = -0.4823265731591e4;
    N8 = 0.40511340542057e6;
    N9 = -0.23855557567849e0;
    N10 = 0.65017534844798e3;
    
    if Ts < 273.15+0.01
        % -100~0.01C//三重点を計算以下は wexler-hyland のシミュレーションプログラム式
        psat = exp(C1 / Ts + C2 + C3 * Ts + C4 * Ts^2 + C5 * Ts^3 + C6 * Ts^4 + C7 * log(Ts)) * P_CONVERT;
    else
        %　~647.096K//臨界温度まで一定とするは IAPWS-IF97 実用国際状態式
        alpha = Ts + N9 / (Ts - N10);
        a2 = alpha * alpha;
        A = a2 + N1 * alpha + N2;
        B = N3 * a2 + N4 * alpha + N5;
        C = N6 * a2 + N7 * alpha + N8;
        psat = (2 * C / (-B + (B * B - 4 * A * C)^0.5))^4 / P_CONVERT;
    end 
    psat = psat*1000; %kPa to Pa
end

== matlab function Integrated_Model/SimpleFCstack/Calc_outlet_humidity/MATLAB Function ==
  data: Ts input; psat output
function psat = sat_vp_pressure(Ts)
    P_CONVERT = 0.001;
    C1 = -5.6745359e3;
    C2 = 6.3925247;
    C3 = -9.6778430e-3;
    C4 = 6.2215701e-7;
    C5 = 2.0747825e-9;
    C6 = -9.4840240e-13;
    C7 = 4.1635019;
    N1 = 0.11670521452767e4;
    N2 = -0.72421316703206e6;
    N3 = -0.17073846940092e2;
    N4 = 0.12020824702470e5;
    N5 = -0.32325550322333e7;
    N6 = 0.14915108613530e2;
    N7 = -0.4823265731591e4;
    N8 = 0.40511340542057e6;
    N9 = -0.23855557567849e0;
    N10 = 0.65017534844798e3;
    
    if Ts < 273.15+0.01
        % -100~0.01C//三重点を計算以下は wexler-hyland のシミュレーションプログラム式
        psat = exp(C1 / Ts + C2 + C3 * Ts + C4 * Ts^2 + C5 * Ts^3 + C6 * Ts^4 + C7 * log(Ts)) * P_CONVERT;
    else
        %　~647.096K//臨界温度まで一定とするは IAPWS-IF97 実用国際状態式
        alpha = Ts + N9 / (Ts - N10);
        a2 = alpha * alpha;
        A = a2 + N1 * alpha + N2;
        B = N3 * a2 + N4 * alpha + N5;
        C = N6 * a2 + N7 * alpha + N8;
        psat = (2 * C / (-B + (B * B - 4 * A * C)^0.5))^4 / P_CONVERT;
    end 
    psat = psat*1000; %kPa to Pa
end

== matlab function Integrated_Model/SimpleFCstack/Calc_outlet_humidity/MATLAB Function1 ==
  data: Ts input; psat output
function psat = sat_vp_pressure(Ts)
    P_CONVERT = 0.001;
    C1 = -5.6745359e3;
    C2 = 6.3925247;
    C3 = -9.6778430e-3;
    C4 = 6.2215701e-7;
    C5 = 2.0747825e-9;
    C6 = -9.4840240e-13;
    C7 = 4.1635019;
    N1 = 0.11670521452767e4;
    N2 = -0.72421316703206e6;
    N3 = -0.17073846940092e2;
    N4 = 0.12020824702470e5;
    N5 = -0.32325550322333e7;
    N6 = 0.14915108613530e2;
    N7 = -0.4823265731591e4;
    N8 = 0.40511340542057e6;
    N9 = -0.23855557567849e0;
    N10 = 0.65017534844798e3;
    
    if Ts < 273.15+0.01
        % -100~0.01C//三重点を計算以下は wexler-hyland のシミュレーションプログラム式
        psat = exp(C1 / Ts + C2 + C3 * Ts + C4 * Ts^2 + C5 * Ts^3 + C6 * Ts^4 + C7 * log(Ts)) * P_CONVERT;
    else
        %　~647.096K//臨界温度まで一定とするは IAPWS-IF97 実用国際状態式
        alpha = Ts + N9 / (Ts - N10);
        a2 = alpha * alpha;
        A = a2 + N1 * alpha + N2;
        B = N3 * a2 + N4 * alpha + N5;
        C = N6 * a2 + N7 * alpha + N8;
        psat = (2 * C / (-B + (B * B - 4 * A * C)^0.5))^4 / P_CONVERT;
    end 
    psat = psat*1000; %kPa to Pa
end

== matlab function Integrated_Model/Simple Compressor/MATLAB Function ==
  data: p input; T input; RH input; yO2 input; M output; R output; cp output; kap output; M_Nmix parameter; M_H2O parameter; M_O2 parameter
%% 湿り空気の状態量計算
function [M, R, cp, kap] = calc_MA_property(p, T, RH, yO2, M_Nmix, M_H2O, M_O2)
    % 湿り空気の物性値計算
    gsprop = GasProperties;
    [M,R,cp,kap] = gsprop.getMAprop(p, T, RH, yO2);
end

%% Calculate saturated vapor pressure [Pa]
function psat = sat_vp_pressure(Ts)
    P_CONVERT = 0.001;
    C1 = -5.6745359e3;
    C2 = 6.3925247;
    C3 = -9.6778430e-3;
    C4 = 6.2215701e-7;
    C5 = 2.0747825e-9;
    C6 = -9.4840240e-13;
    C7 = 4.1635019;
    N1 = 0.11670521452767e4;
    N2 = -0.72421316703206e6;
    N3 = -0.17073846940092e2;
    N4 = 0.12020824702470e5;
    N5 = -0.32325550322333e7;
    N6 = 0.14915108613530e2;
    N7 = -0.4823265731591e4;
    N8 = 0.40511340542057e6;
    N9 = -0.23855557567849e0;
    N10 = 0.65017534844798e3;
    
    if Ts < 273.15+0.01
        % -100~0.01C//三重点を計算以下は wexler-hyland のシミュレーションプログラム式
        psat = exp(C1 / Ts + C2 + C3 * Ts + C4 * Ts^2 + C5 * Ts^3 + C6 * Ts^4 + C7 * log(Ts)) * P_CONVERT;
    else
        %　~647.096K//臨界温度まで一定とするは IAPWS-IF97 実用国際状態式
        alpha = Ts + N9 / (Ts - N10);
        a2 = alpha * alpha;
        A = a2 + N1 * alpha + N2;
        B = N3 * a2 + N4 * alpha + N5;
        C = N6 * a2 + N7 * alpha + N8;
        psat = (2 * C / (-B + (B * B - 4 * A * C)^0.5))^4 / P_CONVERT;
    end 
    psat = psat*1000; %kPa to Pa
end

== matlab function Integrated_Model/SimpleTurbine/MATLAB Function ==
  data: p input; T input; RH input; yO2 input; M output; R output; cp output; kap output; M_Nmix parameter; M_H2O parameter; M_O2 parameter
%% 湿り空気の状態量計算
function [M, R, cp, kap] = calc_MA_property(p, T, RH, yO2, M_Nmix, M_H2O, M_O2)
    % 湿り空気の物性値計算
    gsprop = GasProperties;
    [M,R,cp,kap] = gsprop.getMAprop(p, T, RH, yO2);
end

%% Calculate saturated vapor pressure [Pa]
function psat = sat_vp_pressure(Ts)
    P_CONVERT = 0.001;
    C1 = -5.6745359e3;
    C2 = 6.3925247;
    C3 = -9.6778430e-3;
    C4 = 6.2215701e-7;
    C5 = 2.0747825e-9;
    C6 = -9.4840240e-13;
    C7 = 4.1635019;
    N1 = 0.11670521452767e4;
    N2 = -0.72421316703206e6;
    N3 = -0.17073846940092e2;
    N4 = 0.12020824702470e5;
    N5 = -0.32325550322333e7;
    N6 = 0.14915108613530e2;
    N7 = -0.4823265731591e4;
    N8 = 0.40511340542057e6;
    N9 = -0.23855557567849e0;
    N10 = 0.65017534844798e3;
    
    if Ts < 273.15+0.01
        % -100~0.01C//三重点を計算以下は wexler-hyland のシミュレーションプログラム式
        psat = exp(C1 / Ts + C2 + C3 * Ts + C4 * Ts^2 + C5 * Ts^3 + C6 * Ts^4 + C7 * log(Ts)) * P_CONVERT;
    else
        %　~647.096K//臨界温度まで一定とするは IAPWS-IF97 実用国際状態式
        alpha = Ts + N9 / (Ts - N10);
        a2 = alpha * alpha;
        A = a2 + N1 * alpha + N2;
        B = N3 * a2 + N4 * alpha + N5;
        C = N6 * a2 + N7 * alpha + N8;
        psat = (2 * C / (-B + (B * B - 4 * A * C)^0.5))^4 / P_CONVERT;
    end 
    psat = psat*1000; %kPa to Pa
end

== matlab function Integrated_Model/Turbine Manifold/MATLAB Function ==
  data: p input; T input; RH input; yO2 input; M output; R output; cp output; kap output; M_Nmix parameter; M_H2O parameter; M_O2 parameter
%% 湿り空気の状態量計算
function [M, R, cp, kap] = calc_MA_property(p, T, RH, yO2, M_Nmix, M_H2O, M_O2)
    % 湿り空気の物性値計算
    gsprop = GasProperties;
    [M,R,cp,kap] = gsprop.getMAprop(p, T, RH, yO2);
end

%% Calculate saturated vapor pressure [Pa]
function psat = sat_vp_pressure(Ts)
    P_CONVERT = 0.001;
    C1 = -5.6745359e3;
    C2 = 6.3925247;
    C3 = -9.6778430e-3;
    C4 = 6.2215701e-7;
    C5 = 2.0747825e-9;
    C6 = -9.4840240e-13;
    C7 = 4.1635019;
    N1 = 0.11670521452767e4;
    N2 = -0.72421316703206e6;
    N3 = -0.17073846940092e2;
    N4 = 0.12020824702470e5;
    N5 = -0.32325550322333e7;
    N6 = 0.14915108613530e2;
    N7 = -0.4823265731591e4;
    N8 = 0.40511340542057e6;
    N9 = -0.23855557567849e0;
    N10 = 0.65017534844798e3;
    
    if Ts < 273.15+0.01
        % -100~0.01C//三重点を計算以下は wexler-hyland のシミュレーションプログラム式
        psat = exp(C1 / Ts + C2 + C3 * Ts + C4 * Ts^2 + C5 * Ts^3 + C6 * Ts^4 + C7 * log(Ts)) * P_CONVERT;
    else
        %　~647.096K//臨界温度まで一定とするは IAPWS-IF97 実用国際状態式
        alpha = Ts + N9 / (Ts - N10);
        a2 = alpha * alpha;
        A = a2 + N1 * alpha + N2;
        B = N3 * a2 + N4 * alpha + N5;
        C = N6 * a2 + N7 * alpha + N8;
        psat = (2 * C / (-B + (B * B - 4 * A * C)^0.5))^4 / P_CONVERT;
    end 
    psat = psat*1000; %kPa to Pa
end

== matlab function Integrated_Model/Simple Compressor/Subsystem/MATLAB Function ==
  data: Ts input; psat output
function psat = sat_vp_pressure(Ts)
    P_CONVERT = 0.001;
    C1 = -5.6745359e3;
    C2 = 6.3925247;
    C3 = -9.6778430e-3;
    C4 = 6.2215701e-7;
    C5 = 2.0747825e-9;
    C6 = -9.4840240e-13;
    C7 = 4.1635019;
    N1 = 0.11670521452767e4;
    N2 = -0.72421316703206e6;
    N3 = -0.17073846940092e2;
    N4 = 0.12020824702470e5;
    N5 = -0.32325550322333e7;
    N6 = 0.14915108613530e2;
    N7 = -0.4823265731591e4;
    N8 = 0.40511340542057e6;
    N9 = -0.23855557567849e0;
    N10 = 0.65017534844798e3;
    
    if Ts < 273.15+0.01
        % -100~0.01C//三重点を計算以下は wexler-hyland のシミュレーションプログラム式
        psat = exp(C1 / Ts + C2 + C3 * Ts + C4 * Ts^2 + C5 * Ts^3 + C6 * Ts^4 + C7 * log(Ts)) * P_CONVERT;
    else
        %　~647.096K//臨界温度まで一定とするは IAPWS-IF97 実用国際状態式
        alpha = Ts + N9 / (Ts - N10);
        a2 = alpha * alpha;
        A = a2 + N1 * alpha + N2;
        B = N3 * a2 + N4 * alpha + N5;
        C = N6 * a2 + N7 * alpha + N8;
        psat = (2 * C / (-B + (B * B - 4 * A * C)^0.5))^4 / P_CONVERT;
    end 
    psat = psat*1000; %kPa to Pa
end

== matlab function Integrated_Model/Supply manifold/MATLAB Function ==
  data: p input; T input; RH input; yO2 input; M output; R output; cp output; kap output; M_Nmix parameter; M_H2O parameter; M_O2 parameter
%% 湿り空気の状態量計算
function [M, R, cp, kap] = calc_MA_property(p, T, RH, yO2, M_Nmix, M_H2O, M_O2)
    % 湿り空気の物性値計算
    gsprop = GasProperties;
    [M,R,cp,kap] = gsprop.getMAprop(p, T, RH, yO2);
end

%% Calculate saturated vapor pressure [Pa]
function psat = sat_vp_pressure(Ts)
    P_CONVERT = 0.001;
    C1 = -5.6745359e3;
    C2 = 6.3925247;
    C3 = -9.6778430e-3;
    C4 = 6.2215701e-7;
    C5 = 2.0747825e-9;
    C6 = -9.4840240e-13;
    C7 = 4.1635019;
    N1 = 0.11670521452767e4;
    N2 = -0.72421316703206e6;
    N3 = -0.17073846940092e2;
    N4 = 0.12020824702470e5;
    N5 = -0.32325550322333e7;
    N6 = 0.14915108613530e2;
    N7 = -0.4823265731591e4;
    N8 = 0.40511340542057e6;
    N9 = -0.23855557567849e0;
    N10 = 0.65017534844798e3;
    
    if Ts < 273.15+0.01
        % -100~0.01C//三重点を計算以下は wexler-hyland のシミュレーションプログラム式
        psat = exp(C1 / Ts + C2 + C3 * Ts + C4 * Ts^2 + C5 * Ts^3 + C6 * Ts^4 + C7 * log(Ts)) * P_CONVERT;
    else
        %　~647.096K//臨界温度まで一定とするは IAPWS-IF97 実用国際状態式
        alpha = Ts + N9 / (Ts - N10);
        a2 = alpha * alpha;
        A = a2 + N1 * alpha + N2;
        B = N3 * a2 + N4 * alpha + N5;
        C = N6 * a2 + N7 * alpha + N8;
        psat = (2 * C / (-B + (B * B - 4 * A * C)^0.5))^4 / P_CONVERT;
    end 
    psat = psat*1000; %kPa to Pa
end

== matlab function Integrated_Model/SimpleFCstack/orifiece/calc_phi ==
  data: pin input; phi output; pout input; kap input
function phi = fcn(pin,pout,kap)
    pr = pout/pin;
    p_cr = (2/(kap+1))^(kap/(kap-1))*pin;
    % Judge critical pressure
    if pout < p_cr
        tmp_phi = sqrt(kap*(2/(kap+1))^((kap+1)/(kap-1)));
    else
        % Prevent to become minus values
        a = 1-pr^((kap-1)/kap);
        if a < 0
           a = 0;
        end
        tmp_phi = pr^(1/kap)*sqrt(2*kap/(kap-1)*(a));
    end
    phi = tmp_phi;
end

== matlab function Integrated_Model/Pressure Controller/MATLAB Function ==
  data: Wcr_target input; Ncr_est output; PR_target input; Ncr_table parameter; Wcr_table parameter; PR_table parameter
function Ncr_est = LookUp(Wcr_target,PR_target, Ncr_table, Wcr_table, PR_table)
   Ncr_est = interp2(Wcr_table, PR_table, Ncr_table, Wcr_target, PR_target, 'linear');
end

== matlab function Integrated_Model/Pressure Controller/MATLAB Function1 ==
  data: Wcr output; Wact input; Tin input; pin input; pref parameter; Tref parameter
function Wcr = Wact2Wcr(Wact, Tin,pin, pref, Tref)
    Wcr = Wact * sqrt(Tin/Tref) * pref/pin;
end

== matlab function Integrated_Model/Pressure Controller/MATLAB Function2 ==
  data: Nact output; Ncr input; Tin input; Tref parameter
function Nact = Ncr2Nact(Ncr, Tin, Tref)
    Nact = Ncr * sqrt(Tref/Tin);
end
